simulink model "regcontrol_model_1ph"  (R2018a)
settings: Solver=VariableStepAuto  StartTime=0.0  StopTime=10.0  RelTol=1e-3
values from neighbouring files (symbols this model uses):
  BandWidth = Simulink.Parameter    [start.m]
  BaseVoltage = Simulink.Parameter    [start.m]
  CogenEnabled = false    [regcontrol_emulator.m]    (also in start.m = Simulink.Parameter)
  FPTphase = Simulink.Parameter(FPTphases.DEFAULT)    [regcontrol_emulator.m]    (also in start.m = 1)
  IsReversible = Simulink.Parameter    [start.m]
  LDC_Z = Simulink.Parameter    [start.m]
  MaxTap = 1.10    (= 1.1)    [Transformer.m]
  MinTap = 0.90    (= 0.9)    [Transformer.m]
  PTratio = Simulink.Parameter    [start.m]
  R = 0    [start.m]
  RevBand = Simulink.Parameter    [start.m]
  RevVreg = Simulink.Parameter    [start.m]
  TapLimitPerChange = Simulink.Parameter    [start.m]
  UsingRegulatedBus = Simulink.Parameter    [start.m]
  Vlimit = Simulink.Parameter    [start.m]
  Vreg = Simulink.Parameter    [start.m]
  X = 0    [start.m]
undefined symbols (not defined in the file or in its folder): ControlledTransformerConnection, ControlledTransformerCurrents, ControlledTransformerPowers, ControlledTransformerVoltages, ControlModes, CTRating, IsInverseTime, m, n, NumConductors, NumPhases, PresentTap, RevDelay, revLDC_Z, RevPowerThreshold, revR, revX, TapDelay, TapIncrement, TapWinding, TimeDelay, VTerminal
(part 1 of 2)
settings Model: Creator=Michael Girbino  LastModifiedBy=Michael Girbino
settings CodeAppCC: StateflowObjectComments=on

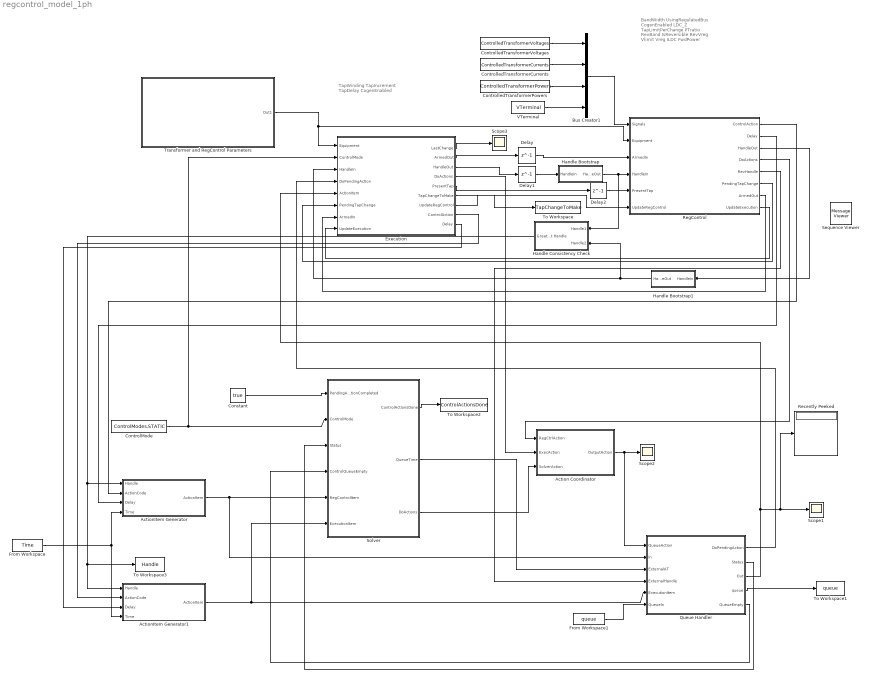
== system regcontrol_model_1ph ==
  note: BandWidth
      | UsingRegulatedBus
      | CogenEnabled
      | LDC_Z
      | TapLimitPerChange
      | PTratio
      | RevBand
      | IsReversible
      | RevVreg
      | Vlimit
      | Vreg
      | ILDC
      | FwdPower
  note: TapWinding
      | TapIncrement
      | TapDelay
      | CogenEnabled
  Action Coordinator : Stateflow chart  TreatAsAtomicUnit=on
  ActionItem Generator : Subsystem
  ActionItem Generator1 : Subsystem
  Bus Creator1 : BusCreator  Inputs=4  OutDataTypeStr=Bus: SignalBus
      settings: InheritFromInputs=off
  Constant : Constant  Value=true  OutDataTypeStr=boolean
  ControlMode : Constant  Value=ControlModes.STATIC  OutDataTypeStr=Enum: ControlModes
  ControlledTransformerCurrents : Constant  Value=ControlledTransformerCurrents
  ControlledTransformerPowers : Constant  Value=ControlledTransformerPowers
  ControlledTransformerVoltages : Constant  Value=ControlledTransformerVoltages
  Delay : Delay  DelayLength=1  InitialCondition=0
  Delay1 : Delay  DelayLength=1  InitialCondition=0
  Delay2 : Delay  DelayLength=1  InitialCondition=0
  Execution : Stateflow chart  TreatAsAtomicUnit=on
  From Workspace : FromWorkspace  VariableName=Time  OutDataTypeStr=double  SampleTime=0
  From Workspace1 : FromWorkspace  VariableName=queue  OutDataTypeStr=fixdt('single', 'DataTypeOverride', 'Off')  SampleTime=0
  Handle Bootstrap : Subsystem
  Handle Bootstrap1 : Subsystem
  Handle Consistency Check : Subsystem
  Queue Handler : Stateflow chart  TreatAsAtomicUnit=on
  Recently Peeked : Display
  RegControl : Stateflow chart  TreatAsAtomicUnit=on
  Scope1 : Scope
  Scope2 : Scope
  Scope3 : Scope
  Sequence Viewer : MessageViewer
  Solver : Stateflow chart  TreatAsAtomicUnit=on
  To Workspace : ToWorkspace  VariableName=TapChangeToMake  SaveFormat=Timeseries  SampleTime=-1
  To Workspace1 : ToWorkspace  VariableName=queue  SaveFormat=Structure With Time  SampleTime=-1
  To Workspace2 : ToWorkspace  VariableName=ControlActionsDone  SaveFormat=Timeseries  SampleTime=-1
  To Workspace3 : ToWorkspace  VariableName=Handle  SaveFormat=Timeseries  SampleTime=-1
  Transformer and RegControl Parameters : Subsystem
  VTerminal : Constant  Value=VTerminal
  wires:
  Queue Handler/5(QueueEmpty) -> Solver/4(ControlQueueEmpty)
  Queue Handler/4(queue) -> To Workspace1/1
  Constant/1 -> Solver/1(PendingActionCompleted)
  Queue Handler/2(Status) -> Solver/3(Status)
  ControlMode/1 -> Execution/2(ControlMode), Solver/2(ControlMode)
  Solver/2(QueueTime) -> Queue Handler/3(ExternalAT)
  Queue Handler/3(Out) -> Recently Peeked/1, Scope1/1, Execution/5(ActionItem)
  ActionItem Generator/1(ActionItem) -> Queue Handler/2(In), Solver/5(RegControlItem)
  Solver/1(ControlActionsDone) -> To Workspace2/1
  RegControl/1(ControlAction) -> ActionItem Generator/2(ActionCode)
  Action Coordinator/1(OutputAction) -> Queue Handler/1(QueueAction), Scope2/1
  Solver/3(DoActions) -> Action Coordinator/3(SolverAction)
  Execution/4(DoActions) -> Action Coordinator/2(ExecAction)
  RegControl/4(DoActions) -> Action Coordinator/1(RegCtrlAction)
  RegControl/2(Delay) -> ActionItem Generator/3(Delay)
  RegControl/3(HandleOut) -> Handle Bootstrap1/1(HandleIn)
  RegControl/5(RevHandle) -> Queue Handler/4(ExternalHandle)
  Execution/3(HandleOut) -> Delay1/1
  Execution/2(ArmedOut) -> Delay/1
  Queue Handler/1(DoPendingAction) -> Execution/4(DoPendingAction)
  Execution/6(TapChangeToMake) -> To Workspace/1
  RegControl/6(PendingTapChange) -> Execution/6(PendingTapChange)
  Execution/1(LastChange) -> Scope3/1
  Handle Consistency Check/1(Greatest Handle) -> To Workspace3/1, ActionItem Generator1/1(Handle), ActionItem Generator/1(Handle)
  Execution/5(PresentTap) -> Delay2/1
  ControlledTransformerVoltages/1 -> Bus Creator1/1
  Transformer and RegControl Parameters/1(Out1) -> Execution/1(Equipment), RegControl/2(Equipment)
  Bus Creator1/1 -> RegControl/1(Signals)
  VTerminal/1 -> Bus Creator1/4
  RegControl/7(ArmedOut) -> Execution/7(ArmedIn)
  ControlledTransformerPowers/1 -> Bus Creator1/3
  ControlledTransformerCurrents/1 -> Bus Creator1/2
  Execution/7(UpdateRegControl) -> RegControl/6(UpdateRegControl)
  RegControl/8(UpdateExecution) -> Execution/8(UpdateExecution)
  Delay/1 -> RegControl/3(ArmedIn)
  Delay1/1 -> Handle Bootstrap/1(HandleIn)
  Delay2/1 -> RegControl/5(PresentTap)
  ActionItem Generator1/1(ActionItem) -> Solver/6(ExecutionItem), Queue Handler/5(ExecutionItem)
  Execution/9(Delay) -> ActionItem Generator1/3(Delay)
  Execution/8(ControlAction) -> ActionItem Generator1/2(ActionCode)
  From Workspace/1 -> ActionItem Generator/4(Time), ActionItem Generator1/4(Time)
  Handle Bootstrap/1(HandleOut) -> RegControl/4(HandleIn), Handle Consistency Check/1(Handle1)
  Handle Bootstrap1/1(HandleOut) -> Handle Consistency Check/2(Handle2), Execution/3(HandleIn)
  From Workspace1/1 -> Queue Handler/6(QueueIn)

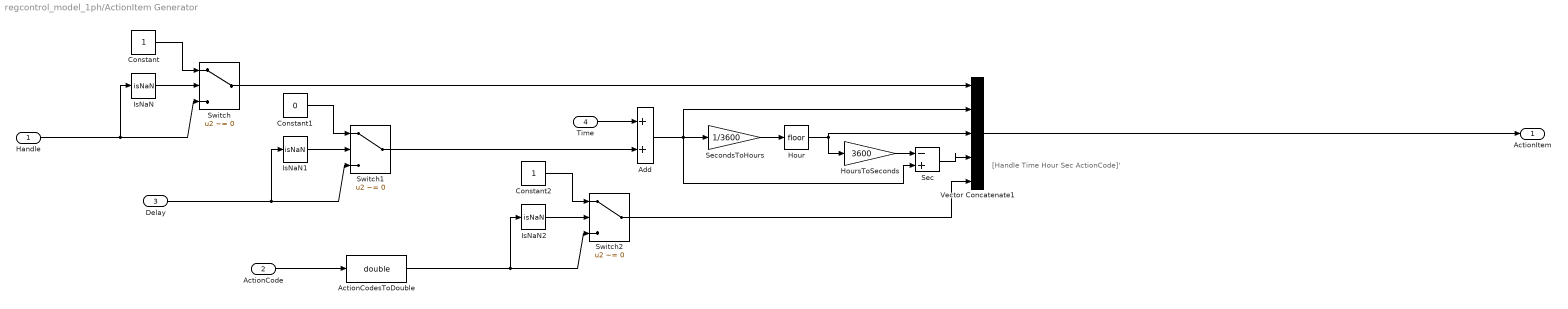
== system regcontrol_model_1ph/ActionItem Generator ==
  note: [Handle Time Hour Sec ActionCode]'
  Handle : Inport
  ActionCode : Inport  Port=2
  Delay : Inport  Port=3
  Time : Inport  Port=4
  ActionCodesToDouble : DataTypeConversion  OutDataTypeStr=double
  Add : Sum
  Constant : Constant
  Constant1 : Constant  Value=0
  Constant2 : Constant
  Hour : Rounding
  HoursToSeconds : Gain  Gain=3600
  IsNaN : RelationalOperator  Operator=isNaN  OutDataTypeStr=boolean  RndMeth=Simplest
  IsNaN1 : RelationalOperator  Operator=isNaN  OutDataTypeStr=boolean  RndMeth=Simplest
  IsNaN2 : RelationalOperator  Operator=isNaN  OutDataTypeStr=boolean  RndMeth=Simplest
  Sec : Sum  Inputs=-+
  SecondsToHours : Gain  Gain=1/3600
  Switch : Switch  Criteria=u2 ~= 0
  Switch1 : Switch  Criteria=u2 ~= 0
  Switch2 : Switch  Criteria=u2 ~= 0
  Vector Concatenate1 : Concatenate  NumInputs=5
  ActionItem : Outport
  wires:
  Add/1 -> Sec/2, SecondsToHours/1, Vector Concatenate1/2
  Hour/1 -> Vector Concatenate1/3, HoursToSeconds/1
  SecondsToHours/1 -> Hour/1
  Vector Concatenate1/1 -> ActionItem/1
  HoursToSeconds/1 -> Sec/1
  Handle/1 -> Switch/3, IsNaN/1
  Sec/1 -> Vector Concatenate1/4
  Time/1 -> Add/1
  ActionCode/1 -> ActionCodesToDouble/1
  IsNaN/1 -> Switch/2
  Constant/1 -> Switch/1
  Switch/1 -> Vector Concatenate1/1
  Delay/1 -> IsNaN1/1, Switch1/3
  IsNaN1/1 -> Switch1/2
  Constant1/1 -> Switch1/1
  Switch1/1 -> Add/2
  ActionCodesToDouble/1 -> Switch2/3, IsNaN2/1
  IsNaN2/1 -> Switch2/2
  Constant2/1 -> Switch2/1
  Switch2/1 -> Vector Concatenate1/5

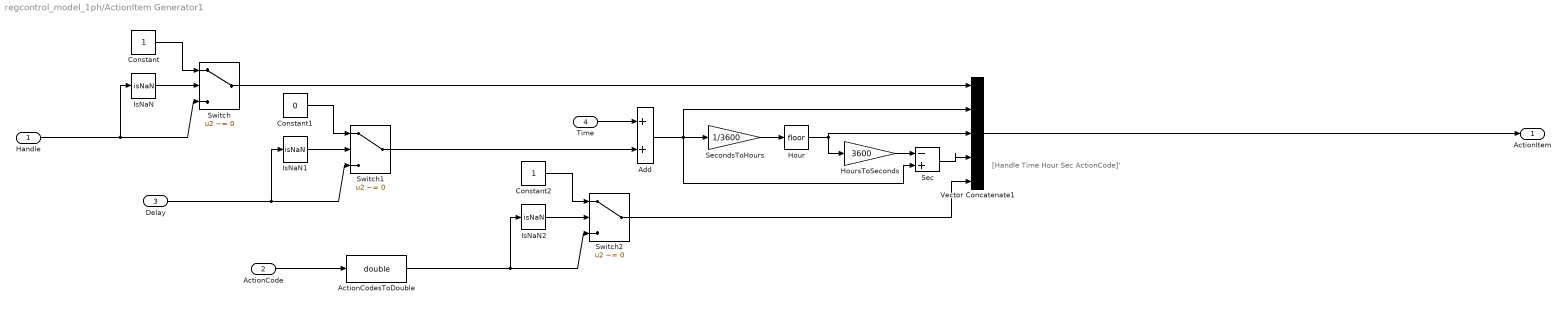
== system regcontrol_model_1ph/ActionItem Generator1 ==
  note: [Handle Time Hour Sec ActionCode]'
  Handle : Inport
  ActionCode : Inport  Port=2
  Delay : Inport  Port=3
  Time : Inport  Port=4
  ActionCodesToDouble : DataTypeConversion  OutDataTypeStr=double
  Add : Sum
  Constant : Constant
  Constant1 : Constant  Value=0
  Constant2 : Constant
  Hour : Rounding
  HoursToSeconds : Gain  Gain=3600
  IsNaN : RelationalOperator  Operator=isNaN  OutDataTypeStr=boolean  RndMeth=Simplest
  IsNaN1 : RelationalOperator  Operator=isNaN  OutDataTypeStr=boolean  RndMeth=Simplest
  IsNaN2 : RelationalOperator  Operator=isNaN  OutDataTypeStr=boolean  RndMeth=Simplest
  Sec : Sum  Inputs=-+
  SecondsToHours : Gain  Gain=1/3600
  Switch : Switch  Criteria=u2 ~= 0
  Switch1 : Switch  Criteria=u2 ~= 0
  Switch2 : Switch  Criteria=u2 ~= 0
  Vector Concatenate1 : Concatenate  NumInputs=5
  ActionItem : Outport
  wires:
  Switch2/1 -> Vector Concatenate1/5
  Constant2/1 -> Switch2/1
  IsNaN2/1 -> Switch2/2
  ActionCodesToDouble/1 -> IsNaN2/1, Switch2/3
  Switch1/1 -> Add/2
  Constant1/1 -> Switch1/1
  IsNaN1/1 -> Switch1/2
  Delay/1 -> Switch1/3, IsNaN1/1
  Switch/1 -> Vector Concatenate1/1
  Constant/1 -> Switch/1
  IsNaN/1 -> Switch/2
  ActionCode/1 -> ActionCodesToDouble/1
  Time/1 -> Add/1
  Sec/1 -> Vector Concatenate1/4
  Handle/1 -> IsNaN/1, Switch/3
  HoursToSeconds/1 -> Sec/1
  Vector Concatenate1/1 -> ActionItem/1
  SecondsToHours/1 -> Hour/1
  Hour/1 -> HoursToSeconds/1, Vector Concatenate1/3
  Add/1 -> Vector Concatenate1/2, SecondsToHours/1, Sec/2

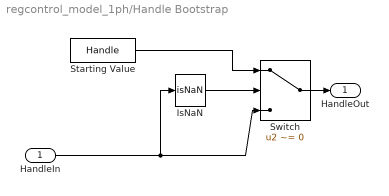
== system regcontrol_model_1ph/Handle Bootstrap ==
  HandleIn : Inport
  IsNaN : RelationalOperator  Operator=isNaN  OutDataTypeStr=boolean  RndMeth=Simplest
  Starting Value : FromWorkspace  VariableName=Handle  OutDataTypeStr=double  SampleTime=0
  Switch : Switch  Criteria=u2 ~= 0
  HandleOut : Outport
  wires:
  IsNaN/1 -> Switch/2
  HandleIn/1 -> Switch/3, IsNaN/1
  Starting Value/1 -> Switch/1
  Switch/1 -> HandleOut/1

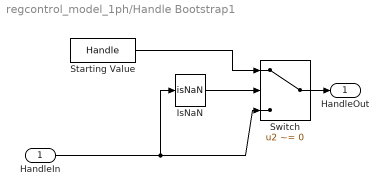
== system regcontrol_model_1ph/Handle Bootstrap1 ==
  HandleIn : Inport
  IsNaN : RelationalOperator  Operator=isNaN  OutDataTypeStr=boolean  RndMeth=Simplest
  Starting Value : FromWorkspace  VariableName=Handle  OutDataTypeStr=double  SampleTime=0
  Switch : Switch  Criteria=u2 ~= 0
  HandleOut : Outport
  wires:
  Switch/1 -> HandleOut/1
  Starting Value/1 -> Switch/1
  HandleIn/1 -> IsNaN/1, Switch/3
  IsNaN/1 -> Switch/2

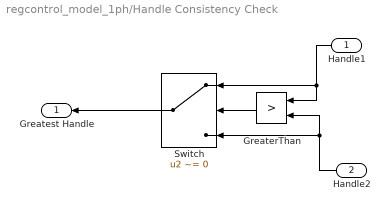
== system regcontrol_model_1ph/Handle Consistency Check ==
  Handle1 : Inport
  Handle2 : Inport  Port=2
  GreaterThan : RelationalOperator  Operator=>  RndMeth=Simplest
  Switch : Switch  Criteria=u2 ~= 0  OutDataTypeStr=double
  Greatest Handle : Outport
  wires:
  Handle2/1 -> GreaterThan/2, Switch/3
  GreaterThan/1 -> Switch/2
  Handle1/1 -> GreaterThan/1, Switch/1
  Switch/1 -> Greatest Handle/1

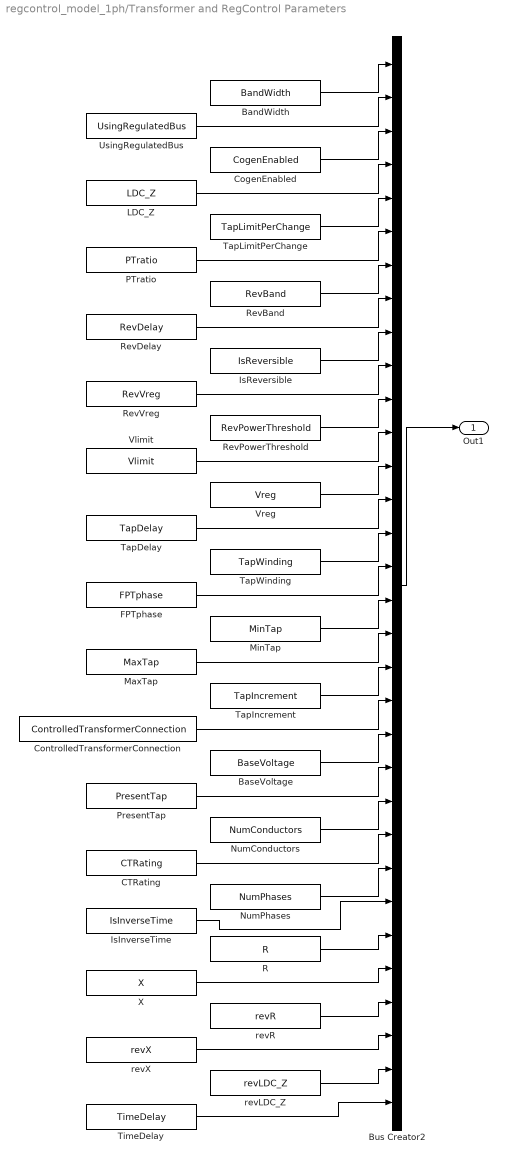
== system regcontrol_model_1ph/Transformer and RegControl Parameters ==
  BandWidth : Constant  Value=BandWidth
  BaseVoltage : Constant  Value=BaseVoltage
  Bus Creator2 : BusCreator  Inputs=32  OutDataTypeStr=Bus: EquipmentBus
      settings: InheritFromInputs=off
  CTRating : Constant  Value=CTRating
  CogenEnabled : Constant  Value=CogenEnabled
  ControlledTransformerConnection : Constant  Value=ControlledTransformerConnection
  FPTphase : Constant  Value=FPTphase
  IsInverseTime : Constant  Value=IsInverseTime
  IsReversible : Constant  Value=IsReversible
  LDC_Z : Constant  Value=LDC_Z
  MaxTap : Constant  Value=MaxTap
  MinTap : Constant  Value=MinTap
  NumConductors : Constant  Value=NumConductors
  NumPhases : Constant  Value=NumPhases
  PTratio : Constant  Value=PTratio
  PresentTap : Constant  Value=PresentTap
  R : Constant  Value=R
  RevBand : Constant  Value=RevBand
  RevDelay : Constant  Value=RevDelay
  RevPowerThreshold : Constant  Value=RevPowerThreshold
  RevVreg : Constant  Value=RevVreg
  TapDelay : Constant  Value=TapDelay
  TapIncrement : Constant  Value=TapIncrement
  TapLimitPerChange : Constant  Value=TapLimitPerChange
  TapWinding : Constant  Value=TapWinding
  TimeDelay : Constant  Value=TimeDelay
  UsingRegulatedBus : Constant  Value=UsingRegulatedBus
  Vlimit : Constant  Value=Vlimit
  Vreg : Constant  Value=Vreg
  X : Constant  Value=X
  revLDC_Z : Constant  Value=revLDC_Z
  revR : Constant  Value=revR
  revX : Constant  Value=revX
  Out1 : Outport
  wires:
  UsingRegulatedBus/1 -> Bus Creator2/2
  BandWidth/1 -> Bus Creator2/1
  TapWinding/1 -> Bus Creator2/15
  TapDelay/1 -> Bus Creator2/14
  Vreg/1 -> Bus Creator2/13
  Vlimit/1 -> Bus Creator2/12
  RevPowerThreshold/1 -> Bus Creator2/11
  RevVreg/1 -> Bus Creator2/10
  IsReversible/1 -> Bus Creator2/9
  RevDelay/1 -> Bus Creator2/8
  RevBand/1 -> Bus Creator2/7
  PTratio/1 -> Bus Creator2/6
  TapLimitPerChange/1 -> Bus Creator2/5
  LDC_Z/1 -> Bus Creator2/4
  CogenEnabled/1 -> Bus Creator2/3
  Bus Creator2/1 -> Out1/1
  FPTphase/1 -> Bus Creator2/16
  MinTap/1 -> Bus Creator2/17
  MaxTap/1 -> Bus Creator2/18
  TapIncrement/1 -> Bus Creator2/19
  ControlledTransformerConnection/1 -> Bus Creator2/20
  BaseVoltage/1 -> Bus Creator2/21
  PresentTap/1 -> Bus Creator2/22
  NumConductors/1 -> Bus Creator2/23
  CTRating/1 -> Bus Creator2/24
  NumPhases/1 -> Bus Creator2/25
  revLDC_Z/1 -> Bus Creator2/31
  revX/1 -> Bus Creator2/30
  revR/1 -> Bus Creator2/29
  X/1 -> Bus Creator2/28
  R/1 -> Bus Creator2/27
  IsInverseTime/1 -> Bus Creator2/26
  TimeDelay/1 -> Bus Creator2/32

== stateflow chart regcontrol_model_1ph/Execution ==
  settings: executeAtInitialization=1
  state Push(CodeVal, DelayVal) [function]
    (default) -> (junction 341) : {ActionCode = CodeVal;
        | Delay = DelayVal;
        | HandleOut = HandleOut + 1;
        | UpdateRegControl.data = ...
        | UpdateActions.HANDLE;
        | send(UpdateRegControl);
        | DoActions.data = QueueActions.PUSH;
        | send(DoActions);}
  state UpdateLocals [parallel]
    settings: executionOrder=2
    state Asleep
      ex: UPDATED = false;
    state UpdateArmed
      en: ArmedOut = ArmedIn;
      ex: UPDATED = true;
    state UpdateHandle
      en:
      if HandleIn > HandleOut
      HandleOut = HandleIn;
      end
      ex: UPDATED = true;
    state UpdatePendingTapChange
      en: LocalPendingTapChange = ...
      PendingTapChange;
      ex: UPDATED = true;
    (default) -> UpdateLocals.Asleep
    UpdateLocals.Asleep -> UpdateHandle [order 3] : UpdateExecution[UpdateExecution.data == ...
        | UpdateActions.HANDLE]
    UpdateLocals.Asleep -> UpdatePendingTapChange [order 1] : UpdateExecution[UpdateExecution.data == ...
        | UpdateActions.PENDING_TAPCHANGE]
    UpdatePendingTapChange -> UpdateLocals.Asleep : [UPDATED]
    UpdateHandle -> UpdateLocals.Asleep : [UPDATED]
    UpdateLocals.Asleep -> UpdateArmed [order 2] : UpdateExecution[UpdateExecution.data == ...
        | UpdateActions.ARMED]
    UpdateArmed -> UpdateLocals.Asleep : [UPDATED]
  state ControlFlow [parallel]
    settings: executionOrder=1
    state Asleep
      ex: AssignInputsToLocals();
      ResetTransitionFlags();
    state MakingTapChange
      state StaticTapChange
        (default) -> (junction 165) : {TapChangeToMake = AtLeastOneTap(LocalPendingTapChange, TapIncrement);
            | % reset to no change = change - 1 program will determin if another is needed:
            | LocalPendingTapChange = 0;
            | UpdateArmed(false);}
      state EventDrivenTapChange
        (default) -> (junction 189) : {[TapChangeToMake LocalPendingTapChange] =...
            |  OneInDirectionOf(LocalPendingTapChange, TapIncrement);
            | UpdatePresentTap(TapChangeToMake);}
        (junction 189) -> (junction 190) [order 1] : [PendingTapChange ~= 0]
        (junction 189) -> (junction 191) [order 2] : {UpdateArmed(false);}
        (junction 190) -> (junction 192) : {Push(ActionCodes.ACTION_TAPCHANGE, TapDelay);}
        (junction 192) -> (junction 191)
      state TimeDrivenTapChange
        (default) -> (junction 200) : {[TapChangeToMake LocalPendingTapChange] =...
            |  OneInDirectionOf(LocalPendingTapChange, TapIncrement);
            | UpdatePresentTap(TapChangeToMake);}
        (junction 200) -> (junction 202) [order 1] : [LocalPendingTapChange ~= 0]
        (junction 200) -> (junction 203) [order 2] : {UpdateArmed(false);}
        (junction 202) -> (junction 201) : {Push(ActionCodes.ACTION_TAPCHANGE, TapDelay);}
        (junction 201) -> (junction 203)
      state MultiRateTapChange
        (default) -> (junction 210) : {[TapChangeToMake, LocalPendingTapChange] =...
            |  OneInDirectionOf(LocalPendingTapChange, TapIncrement);
            | UpdatePresentTap(TapChangeToMake);}
        (junction 210) -> (junction 212) [order 1] : [LocalPendingTapChange ~= 0]
        (junction 210) -> (junction 213) [order 2] : {UpdateArmed(false);}
        (junction 212) -> (junction 211) : {Push(ActionCodes.ACTION_TAPCHANGE, TapDelay);}
        (junction 211) -> (junction 213)
      state Finished
        en: EXIT_TAPCHANGE = true;
      (default) -> (junction 132)
      (junction 132) -> (junction 133) [order 1] : % Check to make sure control has not reset:
          | [LocalPendingTapChange == 0]
      (junction 132) -> (junction 163) [order 2]
      (junction 133) -> (junction 135) : {UpdateArmed(false);}
      (junction 163) -> StaticTapChange [order 1] : [ControlMode == ControlModes.STATIC]
      (junction 163) -> (junction 167) [order 2]
      StaticTapChange -> (junction 170)
      (junction 167) -> EventDrivenTapChange [order 1] : [ControlMode == ControlModes.EVENTDRIVEN]
      (junction 167) -> (junction 171) [order 2]
      EventDrivenTapChange -> (junction 169)
      (junction 169) -> (junction 170)
      (junction 170) -> (junction 174)
      (junction 171) -> TimeDrivenTapChange [order 1] : [ControlMode == ControlModes.TIMEDRIVEN]
      (junction 171) -> (junction 175) [order 2]
      TimeDrivenTapChange -> (junction 173)
      (junction 173) -> (junction 174)
      (junction 174) -> (junction 178)
      (junction 175) -> MultiRateTapChange [order 1] : [ControlMode == ControlModes.MULTIRATE]
      (junction 175) -> (junction 179) [order 2]
      (junction 178) -> (junction 180)
      MultiRateTapChange -> (junction 357)
      (junction 357) -> (junction 179)
      (junction 180) -> (junction 357)
      (junction 179) -> ControlFlow.MakingTapChange.Finished
      (junction 135) -> ControlFlow.MakingTapChange.Finished
    state Reversing
      state FlipCogen
        (default) -> (junction 252)
        (junction 252) -> (junction 253) [order 1] : [InCogenMode]
        (junction 252) -> (junction 254) [order 2] : {InCogenMode = true;}
        (junction 253) -> (junction 255) : {InCogenMode = false;}
        (junction 255) -> (junction 254)
      state FlipReverse
        (default) -> (junction 263)
        (junction 263) -> (junction 264) [order 1] : [InReverseMode]
        (junction 263) -> (junction 265) [order 2] : {InReverseMode = true;}
        (junction 264) -> (junction 266) : {InReverseMode = false;}
        (junction 266) -> (junction 265)
      state Finished
        en: EXIT_REVERSE = true;
      (default) -> (junction 229)
      (junction 229) -> (junction 230) [order 1] : [ReversePending]
      (junction 229) -> (junction 231) [order 2]
      (junction 230) -> (junction 242)
      (junction 242) -> (junction 238) [order 1] : [CogenEnabled]
      (junction 242) -> FlipReverse [order 2]
      (junction 238) -> FlipCogen : % Cogen mode takes precedence if present
      FlipCogen -> (junction 245)
      FlipReverse -> (junction 240)
      (junction 245) -> (junction 240)
      (junction 240) -> (junction 232) : {ReversePending = false;}
      (junction 232) -> (junction 231)
      (junction 231) -> ControlFlow.Reversing.Finished
    state Finished
    (default) -> ControlFlow.Asleep
    ControlFlow.Finished -> ControlFlow.Asleep
    ControlFlow.Asleep -> (junction 115) : DoPendingAction
    (junction 115) -> MakingTapChange [order 1] : [Code == ActionCodes.ACTION_TAPCHANGE]
    (junction 115) -> (junction 119) [order 2]
    MakingTapChange -> (junction 117) : [EXIT_TAPCHANGE]
    (junction 117) -> (junction 118)
    (junction 118) -> (junction 122)
    (junction 119) -> Reversing [order 1] : [Code == ActionCodes.ACTION_REVERSE]
    (junction 119) -> (junction 123) [order 2]
    Reversing -> (junction 122)
    (junction 122) -> (junction 124) : [EXIT_REVERSE]
    (junction 124) -> (junction 123)
    (junction 123) -> ControlFlow.Finished
  state AssignInputsToLocals [function]
    note: TapWinding
        | TapIncrement
        | TapDelay
        | CogenEnabled
    (default) -> (junction 375) : {% From Script:
        | TapWinding = Equipment.TapWinding;
        | TapIncrement = Equipment.TapIncrement;
        | TapDelay = Equipment.TapDelay;
        | CogenEnabled = Equipment.CogenEnabled;
        | PresentTap = Equipment.PresentTap;
        | TapLimitPerChange = Equipment.TapLimitPerChange;
        | % From the ControlQueue:
        | Code = ...
        | uint8(ActionItem(NewCtrlQueueFields.ActionCode));
        | % PendingTapChange:
        | % LocalPendingTapChange = PendingTapChange;
        | %ArmedOut = ArmedIn;
        | }
  state ChangeToMake = AtLeastOneTap(ProposedChange, Increment) [function]
    note: Called in STATIC mode
        | Changes 70% of the way but at least one tap, subject to maximum allowable tap change
    (default) -> (junction 283) : {NumTaps = floor(0.7 * abs(ProposedChange)/Increment);}
    (junction 283) -> (junction 284) [order 1] : [NumTaps == 0]
    (junction 283) -> (junction 285) [order 2]
    (junction 284) -> (junction 286) : {NumTaps = 1.0;} % At least 1 tap
    (junction 286) -> (junction 285)
    (junction 285) -> (junction 293)
    (junction 293) -> (junction 290) [order 1] : [NumTaps > TapLimitPerChange]
    (junction 293) -> (junction 294) [order 2]
    (junction 290) -> (junction 295) : {NumTaps = double(TapLimitPerChange);} % Bound by maximum
    (junction 295) -> (junction 294)
    (junction 294) -> (junction 302) : {LastChange = NumTaps;}
    (junction 302) -> (junction 303) [order 1] : % Check sign on change:
        | [ProposedChange > 0]
    (junction 302) -> (junction 304) [order 2] : {ChangeToMake = -1*double(NumTaps)*Increment;
        | LastChange = -1*NumTaps;}
    (junction 303) -> (junction 305) : {ChangeToMake =...
        |  double(NumTaps)*Increment;}
    (junction 305) -> (junction 304)
    (junction 304) -> (junction 306)
  state ResetTransitionFlags [function]
    (default) -> (junction 377) : {EXIT_TAPCHANGE = false;
        | EXIT_REVERSE = false;}
  state [ChangeToMake, NewProposedChange] = OneInDirectionOf(ProposedChange, Increment) [function]
    note: Computes the amount of one tap change in the direction of the pending tapchange
        | Automatically decrements the proposed change by that amount
    (default) -> (junction 318) : {LastChange = 0;}
    (junction 318) -> (junction 319) [order 1] : [ProposedChange > 0]
    (junction 318) -> (junction 320) [order 2] : {ChangeToMake = -1*Increment;
        | LastChange = -1;
        | NewProposedChange = ProposedChange + Increment;}
    (junction 319) -> (junction 321) : {ChangeToMake = Increment;
        | LastChange = 1;
        | NewProposedChange =...
        |  ProposedChange - Increment;}
    (junction 321) -> (junction 320)
    (junction 320) -> (junction 329)
    (junction 329) -> (junction 330) [order 1] : [abs(NewProposedChange) < 0.9*Increment]
    (junction 329) -> (junction 331) [order 2]
    (junction 330) -> (junction 332) : {NewProposedChange = 0;}
    (junction 332) -> (junction 331)
    (junction 331) -> (junction 333)
  state UpdatePresentTap(Change) [function]
    (default) -> (junction 415) : {
        | PresentTap = PresentTap + Change;
        | UpdateRegControl.data = ...
        | UpdateActions.PRESENT_TAP;
        | send(UpdateRegControl);
        | }
  state UpdateArmed(NewArmed) [function]
    (default) -> (junction 419) : {
        | ArmedOut = NewArmed;
        | UpdateRegControl.data = ...
        | UpdateActions.ARMED;
        | send(UpdateRegControl);
        | }
  data: CodeVal function_input; DelayVal function_input; ProposedChange function_input; Increment function_input; ChangeToMake function_output; NumTaps local double; ProposedChange function_input; Increment function_input; ChangeToMake function_output; NewProposedChange function_output; Change function_input; NewArmed function_input; Equipment input Bus: EquipmentBus; LastChange output double; ControlMode input Enum: ControlModes; HandleIn input double; ArmedOut output boolean =false; HandleOut output double =0; DoActions output Enum: QueueActions; PresentTap output double; EXIT_REVERSE local boolean; InReverseMode local boolean; EXIT_TAPCHANGE local boolean; ReversePending local boolean; InCogenMode local boolean; DoPendingAction input boolean; TapWinding local uint8; TapIncrement local double; TapDelay local double; CogenEnabled local boolean =false; Code local uint8; ActionItem input double size=[1 5]; TapChangeToMake output double; PendingTapChange input double size=[1]; LocalPendingTapChange local double =double(0); ArmedIn input boolean; TapLimitPerChange local uint8 =uint8(16); UpdateRegControl output Enum: UpdateActions; UpdateExecution input Enum: UpdateActions; UPDATED local boolean =false; ControlAction output Enum: ActionCodes; Delay output double =0

== stateflow chart regcontrol_model_1ph/Solver ==
  state ControlFlow
    note: Static
        | - placeholder QueueTime
        | - DoNearestActions
    note: Event-driven
        | - QueueTime is current time
        | - DoNearestActions
    note: Time-driven
        | - QueueTime is current time
        | - DoActions
    note: Multirate
        | - QueueTime is current time
        | - DoMultiRate
    (default) -> (junction 25) : {TimeInSec = RegControlItem(NewCtrlQueueFields.Time);}
    (junction 25) -> (junction 26) [order 1] : [ControlMode == ControlModes.STATIC]
    (junction 25) -> (junction 29) [order 2]
    (junction 26) -> (junction 54)
    (junction 54) -> (junction 55) [order 1] : [LocalControlQueueEmpty]
        | % execute nearest set of control actions, but leave time where it is
    (junction 54) -> (junction 56) [order 2] : {QueueTime = 0; %[0 0] xHour, xSec
        | DoActions.data = QueueActions.DO_NEAREST_ACTIONS;
        | send(DoActions);
        | % ignores time advancement
        | }
    (junction 55) -> (junction 57) : {ControlActionsDone = true;}
    (junction 57) -> (junction 56)
    (junction 56) -> (junction 27)
    (junction 27) -> (junction 28)
    (junction 28) -> (junction 32)
    (junction 29) -> (junction 30) [order 1] : [ControlMode == ControlModes.EVENTDRIVEN]
        | % execute nearest set of control actions and advance time to that time
    (junction 30) -> (junction 65) : {QueueTime = TimeInSec; %xHour, xSec
        | DoActions.data = QueueActions.DO_NEAREST_ACTIONS;
        | send(DoActions);}
    (junction 29) -> (junction 33) [order 2]
    (junction 65) -> (junction 66) [order 1] : [~PendingActionCompleted]
    (junction 65) -> (junction 67) [order 2]
    (junction 66) -> (junction 68) : {ControlActionsDone = true;
        | % advances time to the next event
        | }
    (junction 68) -> (junction 67)
    (junction 67) -> (junction 31)
    (junction 31) -> (junction 32)
    (junction 32) -> (junction 36)
    (junction 33) -> (junction 34) [order 1] : [ControlMode == ControlModes.TIMEDRIVEN]
        |  % Do all actions having and action time <= specified time
    (junction 33) -> (junction 37) [order 2]
    (junction 34) -> (junction 78) : {QueueTime = TimeInSec; %xHour, xSec
        | DoActions.data = QueueActions.DO_ACTIONS;
        | send(DoActions);}
    (junction 78) -> (junction 80) [order 1] : [~PendingActionCompleted]
    (junction 78) -> (junction 79) [order 2]
    (junction 80) -> (junction 82) : {ControlActionsDone = true;
        | }
    (junction 82) -> (junction 79)
    (junction 79) -> (junction 35)
    (junction 35) -> (junction 36)
    (junction 36) -> (junction 40)
    (junction 37) -> (junction 38) [order 1] : [ControlMode == ControlModes.MULTIRATE]
        |  % Execute the nearest set of control actions, but leave time where it is
    (junction 37) -> (junction 41) [order 2]
    (junction 38) -> (junction 91) : {QueueTime =TimeInSec; %xHour, xSec
        | DoActions.data = QueueActions.DO_MULTIRATE;
        | send(DoActions);}
    (junction 91) -> (junction 88) [order 1] : [~PendingActionCompleted]
    (junction 91) -> (junction 87) [order 2]
    (junction 88) -> (junction 92) : {ControlActionsDone = true;
        | }
    (junction 92) -> (junction 87)
    (junction 87) -> (junction 39)
    (junction 39) -> (junction 40)
    (junction 40) -> (junction 42)
    (junction 42) -> (junction 41)
    (junction 41) -> (junction 43)
  state QueueEmptyCase
    en: LocalControlQueueEmpty = true;
  (default) -> ControlFlow
  QueueEmptyCase -> ControlFlow
  ControlFlow -> QueueEmptyCase : ControlQueueEmpty
  data: ControlActionsDone output boolean; QueueTime output double; DoActions output Enum: QueueActions; PendingActionCompleted input boolean; ControlMode input Enum: ControlModes; ii local double =0; Status input Enum: Statuses; LocalControlQueueEmpty local boolean =false; ControlQueueEmpty input boolean; TimeInSec local double; RegControlItem input double size=[5 1]; ExecutionItem input double size=[5 1]

== stateflow chart regcontrol_model_1ph/Action Coordinator ==
  state Asleep
  state SendingRegCtrlAction
    en:OutputAction.data = ...
    RegCtrlAction.data;
    send(OutputAction);
  state SendingSolverAction
    en:OutputAction.data = ...
    SolverAction.data;
    send(OutputAction);
  state SendingExecAction
    en:OutputAction.data = ...
    ExecAction.data;
    send(OutputAction);
  (default) -> Asleep
  Asleep -> SendingRegCtrlAction [order 1] : RegCtrlAction
  Asleep -> SendingSolverAction [order 3] : SolverAction
  SendingSolverAction -> Asleep
  SendingRegCtrlAction -> Asleep
  Asleep -> SendingExecAction [order 2] : ExecAction
  SendingExecAction -> Asleep
  data: RegCtrlAction input Enum: QueueActions; ExecAction input Enum: QueueActions; SolverAction input Enum: QueueActions; OutputAction output Enum: QueueActions

== stateflow chart regcontrol_model_1ph/Queue Handler ==
  settings: enableNonTerminalStates=1
  state Executive [parallel]
    settings: executionOrder=1
    state Asleep
      ex: Status.data = Statuses.READY; % reset status
      INTERNAL_DONE = false;
      EXECUTIVE_DONE = false;
    state DoNearestActions
      state WaitOnPeek
        en: send(QUEUE_PEEK, Internal);
      state WaitOnPop
        en: send(QUEUE_POP, Internal);
      state ErrorNoItems
        en: Status.data = ...
        Statuses.ERROR;
        send(Status);
      (default) -> (junction 302) : % do only those actions with the same delay time as the first action time return time
          | {q_len_initial = GetQueueSize;
          | PendingActionsCompleted = false; % local for now
          | }
      (junction 302) -> (junction 315) [order 1] : [q_len_initial > 0]
      (junction 302) -> Executive.DoNearestActions.ErrorNoItems [order 2]
      (junction 315) -> WaitOnPeek : {INTERNAL_DONE = false;
          | ActionTime = uint8(ExternalAT); % peek with given AT
          | }
      (junction 301) -> (junction 331) [order 1] : [jj <= q_len_initial]
      (junction 331) -> Executive.DoNearestActions.WaitOnPop : {INTERNAL_DONE = false;}
      WaitOnPeek -> (junction 301) : [INTERNAL_DONE]
          | {ActionTime = uint8(Out(QF.Time));
          | QHour = Out(QF.Hour);
          | QSec = Out(QF.Sec);
          | jj = 1;}
      Executive.DoNearestActions.WaitOnPop -> (junction 299) : [INTERNAL_DONE]
          | %send(DoPendingAction);
      (junction 299) -> (junction 301) : {jj = jj + 1;}
      (junction 301) -> (junction 305) [order 2]
      Executive.DoNearestActions.ErrorNoItems -> (junction 300)
      (junction 305) -> (junction 300)
      (junction 300) -> (junction 298) : {EXECUTIVE_DONE = true;}
    state DoAllActions
      state WaitOnPop
        en: send(QUEUE_POP, Internal);
      state ErrorNoItems
        en: Status.data = ...
        Statuses.ERROR;
        send(Status);
      state Finished
      (default) -> (junction 322) : {q_len_initial = GetQueueSize;}
      (junction 322) -> (junction 321) [order 1] : [q_len_initial ~= 0]
      (junction 322) -> Executive.DoAllActions.ErrorNoItems [order 2]
      (junction 321) -> (junction 326) : {ActionTime = uint8(ExternalAT);
          | jj = 1;}
      (junction 326) -> (junction 316) [order 1] : [jj <= q_len_initial]
      (junction 316) -> Executive.DoAllActions.WaitOnPop : {INTERNAL_DONE = false;}
      (junction 314) -> (junction 326) : {jj = jj + 1;}
      (junction 326) -> (junction 312) [order 2]
      Executive.DoAllActions.WaitOnPop -> (junction 314) : [INTERNAL_DONE]
          | %send(DoPendingAction);
      Executive.DoAllActions.ErrorNoItems -> (junction 324)
      (junction 312) -> (junction 324)
      (junction 324) -> Finished : {EXECUTIVE_DONE = true;}
    state Pushing
      en: send(QUEUE_PUSH, Internal);
    state DeletingByHandle
      en: send(QUEUE_DELETE, Internal);
    state Peeking
      en: send(QUEUE_PEEK, Internal);
    state Popping
      en: send(QUEUE_POP, Internal);
    state ReadyAgain
      Status.data = Statuses.READY;
      send(Status);
    Executive.Asleep -> Executive.DeletingByHandle [order 6] : QueueAction[QueueAction.data == ...
        | QueueActions.DELETE]
    Executive.Asleep -> Executive.Peeking [order 5] : QueueAction[QueueAction.data == ...
        | QueueActions.PEEK]
    Executive.Asleep -> Executive.Popping [order 4] : QueueAction[QueueAction.data == ...
        | QueueActions.POP]
    (default) -> Executive.Asleep
    Executive.Asleep -> Executive.Pushing [order 3] : QueueAction[QueueAction.data == ...
        | QueueActions.PUSH]
    Executive.Asleep -> DoAllActions [order 2] : QueueAction[QueueAction.data == ...
        | QueueActions.DO_ALL_ACTIONS]
    ReadyAgain -> Executive.Asleep
    Executive.Asleep -> DoNearestActions [order 1] : QueueAction[QueueAction.data == DO_NEAREST_ACTIONS]
    Executive.Pushing -> ReadyAgain : [INTERNAL_DONE]
    Executive.Popping -> ReadyAgain : [INTERNAL_DONE]
    Executive.DeletingByHandle -> ReadyAgain : [INTERNAL_DONE]
    Executive.Peeking -> ReadyAgain : [INTERNAL_DONE]
    DoAllActions -> ReadyAgain : [EXECUTIVE_DONE]
    DoNearestActions -> ReadyAgain : [EXECUTIVE_DONE]
  state Internal [parallel]
    settings: executionOrder=2
    state Asleep
    state Popping
      (default) -> (junction 163) : % delete from beginning, t<= ActionTime:
          | {q_len = GetQueueSize;
          | ii = 1;
          | }
      (junction 163) -> (junction 169) [order 1] : [ii <= q_len]
      (junction 169) -> (junction 157)
      (junction 157) -> (junction 158) [order 1] : [GetElemTime(ii) <= ActionTime]
      (junction 157) -> (junction 164) [order 2]
      (junction 158) -> (junction 159) : {Out = GetElem(ii);
          | ReduceQueue(ii);
          | send(DoPendingAction);}
          | % break
      (junction 164) -> (junction 163) : {ii = ii + 1;}
      (junction 163) -> (junction 165) [order 2]
      (junction 159) -> (junction 165)
      (junction 165) -> (junction 640)
      (junction 640) -> (junction 641) [order 1] : [QueueEmpty.data == true]
      (junction 640) -> (junction 642) [order 2]
      (junction 641) -> (junction 643) : {send(QueueEmpty);}
      (junction 643) -> (junction 642)
      (junction 642) -> (junction 644) : {INTERNAL_DONE = true;}
    state DeletingByHandle
      (default) -> (junction 664) : % delete from beginning, t<= ActionTime:
          | {q_len = GetQueueSize;
          | ii = 1;
          | }
      (junction 664) -> (junction 671) [order 1] : [ii <= q_len]
      (junction 671) -> (junction 670)
      (junction 670) -> (junction 665) [order 1] : [GetElemHandle(ii) == uint8(ExternalHandle)]
      (junction 670) -> (junction 663) [order 2]
      (junction 665) -> (junction 660) : {Out = GetElem(ii);
          | ReduceQueue(ii);}
          | % break
      (junction 663) -> (junction 664) : {ii = ii + 1;}
      (junction 664) -> (junction 668) [order 2]
      (junction 660) -> (junction 668)
      (junction 668) -> (junction 666)
      (junction 666) -> (junction 658) [order 1] : [QueueEmpty.data == true]
      (junction 666) -> (junction 661) [order 2]
      (junction 658) -> (junction 667) : {send(QueueEmpty);}
      (junction 667) -> (junction 661)
      (junction 661) -> (junction 655) : {INTERNAL_DONE = true;}
    state Pushing
      (default) -> (junction 136) : % insert into queue right before item of greater or equal execution time
          | {q_cand = ChooseItem;
          | q_len = GetQueueSize; %size(queue, 3);
          | ii = 1;
          | }
      (junction 136) -> (junction 134) [order 1] : [ii <= q_len]
      (junction 134) -> (junction 145)
      (junction 145) -> (junction 146) [order 1] : [q_cand(1,QF.Time) <= GetElemTime(ii)]
      (junction 145) -> (junction 137) [order 2]
      (junction 146) -> (junction 148) : {
          | ExpandQueue(ii);}
          | % break
      (junction 137) -> (junction 136) : {ii = ii + 1;}
      (junction 136) -> (junction 138) [order 2] : {ExpandQueue(q_len+1);}
      (junction 148) -> (junction 138)
      (junction 138) -> (junction 151) : %{send(DONE_PUSHING, Executive.Pushing);}
          | {INTERNAL_DONE = true;}
    state Peeking
      (default) -> (junction 181) : % pop without deletion
          | {q_len = GetQueueSize;
          | ii = 1;
          | }
      (junction 181) -> (junction 187) [order 1] : [ii <= q_len]
      (junction 187) -> (junction 175)
      (junction 175) -> (junction 176) [order 1] : [GetElemTime(ii) <= ActionTime]
      (junction 175) -> (junction 182) [order 2]
      (junction 176) -> (junction 177) : {Out = GetElem(ii);}
          | % break
      (junction 182) -> (junction 181) : {ii = ii + 1;}
      (junction 181) -> (junction 183) [order 2]
      (junction 177) -> (junction 183)
      (junction 183) -> (junction 180) : {INTERNAL_DONE = true;}
    (default) -> Internal.Asleep
    Internal.Asleep -> Internal.Pushing [order 1] : QUEUE_PUSH
    Internal.Pushing -> Internal.Asleep : [INTERNAL_DONE]
    Internal.Asleep -> Internal.Popping [order 2] : QUEUE_POP
    Internal.Popping -> Internal.Asleep : [INTERNAL_DONE]
    Internal.Asleep -> Internal.Peeking [order 3] : QUEUE_PEEK
    Internal.Peeking -> Internal.Asleep : [INTERNAL_DONE]
    Internal.Asleep -> Internal.DeletingByHandle [order 4] : QUEUE_DELETE
    Internal.DeletingByHandle -> Internal.Asleep : [INTERNAL_DONE]
  state Item = ChooseItem [function]
    (default) -> (junction 716) : % Choose item with biggest handle (most recent):
    (junction 716) -> (junction 717) [order 1] : [In(QF.Handle) > ExecutionItem(QF.Handle)]
    (junction 717) -> (junction 719) : {Item = In';}
    (junction 716) -> (junction 718) [order 2] : {Item = ExecutionItem';}
    (junction 719) -> (junction 718)
    (junction 718) -> (junction 720)
  state QF % Queue Fields [group]
  state qs = GetQueueSize [function]
    (default) -> (junction 686) : {[qs, QueueEmpty.data] = mlGetQueueSize;}
  data: Item function_output; Handle local double =1; Time local double =2; Hour local double =3; Sec local double =4; qs function_output; depth function_input; h function_output; qs function_output; qe_data function_output; depth function_input; et function_output; elem function_output; depth function_input; depth function_input; depth function_input; DoPendingAction output boolean =true; QueueAction input Enum: QueueActions; Status output Enum: Statuses; Out output double size=[1 5]; queue output double size=[1 5 1]; q_len local double =0; PendingActionsCompleted local boolean =false; QHour local double; QSec local double; q_cand local double size=[1 5]; In input double size=[5 1]; qwriteflag local boolean =false; ii local uint8; jj local uint8; q_len_initial local double; EXECUTIVE_DONE local boolean =false; INTERNAL_DONE local boolean =false;; ExternalAT input double =100; ActionTime local uint8; QueueEmpty output boolean =false; ExternalHandle input uint8 size=1; ExecutionItem input double size=[5 1]; QueueIn input double size=[1 5 1]
  events: QUEUE_POP local FUNCTION_CALL_EVENT; QUEUE_PUSH local FUNCTION_CALL_EVENT; QUEUE_PEEK local FUNCTION_CALL_EVENT; QUEUE_DELETE local FUNCTION_CALL_EVENT
  function h = GetElemHandle(depth):
    | function h = GetElemHandle(depth)
    |     hh = zeros(1,1);
    |     if ~isempty(queue)
    |         hh = queue(1,QF.Handle,ii);        
    |     end
    |     h = cast(hh, 'uint8'); % for comparison with ExternalHandle
    | end
  function [qs, qe_data] = mlGetQueueSize:
    | function [qs, qe_data] = mlGetQueueSize
    | %     coder.extrinsic('exist');
    | %     eq = zeros(1,1,'double');
    | %     eq = exist('queue');
    | %     if eq == 1 && ~isempty(queue)
    | %         qs = size(queue, 3);
    | %     else % eq ~= 1 || size == 0
    | %         qs = 0;
    | %     end
    |     if ~qwriteflag % can't read intial value of empty queue, so depend on flag
    |         if exist QueueIn
    |             queue = QueueIn;
    |         else
    |             queue = zeros(1,5);
    |         end
    |         qs = 0;
    |         qe_data = true;
    |         %QueueEmpty.data = true;
    |         qwriteflag = true;
    |     elseif isequal(queue,zeros(1,5)) % case of empty queue (still 1 element)
    |         qs = 0;
    |         qe_data = true;
    |         %QueueEmpty.data = true;
    |     else
    |         qs = size(queue,3);
    |         qe_data = false;
    |         %QueueEmpty.data = false;
    |     end
    | end
  function et = GetElemTime(depth):
    | function et = GetElemTime(depth)
    |     et = zeros(1,1);
    |     if ~isempty(queue)
    |         et = queue(1,QF.Time,ii);
    |     else
    |     end
    | end
  function elem = GetElem(depth):
    | function elem = GetElem(depth)
    |     elem = zeros(1,5);
    |     elem(1,:) = queue(:,:,depth);
    | end
  function ExpandQueue(depth):
    | function ExpandQueue(depth)
    |     rhs = queue(:,:,depth:q_len); % the RHS of the queue
    |     bigger = zeros(1,5,q_len+1);
    |     bigger(:,:,1:(depth-1)) = queue(:,:,1:(depth-1)); % copy LHS
    |     bigger(:,:,depth) = q_cand; % inserting element at end of LHS
    |     %queue(:,:,depth) = q_cand; 
    |     bigger(:,:, (depth+1):(q_len+1)) = rhs; % tack on RHS again
    |     queue = bigger;
    | end
  function ReduceQueue(depth):
    | function ReduceQueue(depth)
    |     rhs = queue(:,:,(depth+1):q_len); % excluding element at depth
    |     smaller = zeros(1,5,q_len-1);
    |     smaller(:,:,1:(depth-1)) = queue(:,:,1:(depth-1)); % lhs, excl. depth
    |     smaller(:,:,depth:(q_len-1)) = rhs; % tack on rhs
    |     queue = smaller;
    | end
